simulink model "adrc"  (R2017a)
settings: Solver=FixedStepAuto  StartTime=0.0  StopTime=4  FixedStep=1/30e3  RelTol=1e-3
undefined symbols (not defined in the file): adrc_lib, DiscIntNeverNeededParam, DistObs, h, J, K, Kf, L, R
libraries: simulink_extras x5
settings Model: Creator=uids8840  LastModifiedBy=root

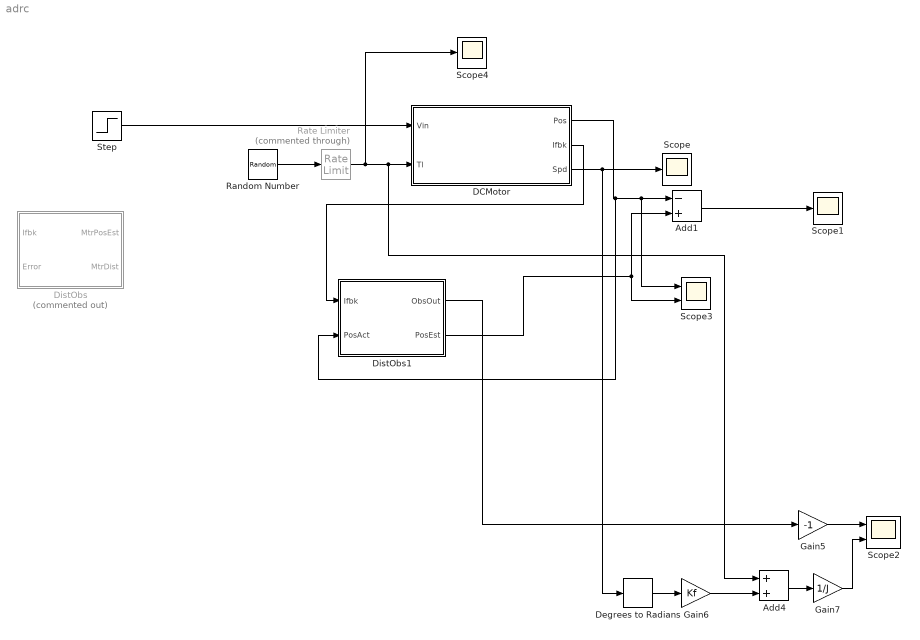
== system adrc ==
  Add1 : Sum  Inputs=-+
  Add4 : Sum
  DCMotor : Subsystem
  Degrees to Radians : simulink_extras/Transformations/Degrees to Radians
  DistObs : Subsystem  Commented=on  SystemSampleTime=1e-3
  DistObs1 : Subsystem  AncestorBlock=adrc_lib/DistObs  TreatAsAtomicUnit=on  SystemSampleTime=1/30e3  mask{k0=-800, k1=-25, k2=-1/4, Jest=J, Kest=K, ts=1/30e3}
      mask prompts: Jest "Motor Inertia [J]"; Kest "Motor Constant [K]"; ts "Execution rate [s]"
  Gain5 : Gain  Gain=-1
  Gain6 : Gain  Gain=Kf
  Gain7 : Gain  Gain=1/J
  Random Number : RandomNumber  Mean=0.03  SampleTime=0.1
  Rate Limiter : RateLimiter  Commented=through  RisingSlewLimit=1e-4  FallingSlewLimit=-1e-4  SampleTimeMode=inherited
  Scope : Scope
  Scope1 : Scope
  Scope2 : Scope  NumInputPorts=2
  Scope3 : Scope  NumInputPorts=2
  Scope4 : Scope
  Step : Step  Time=0.1  After=24  SampleTime=0
  wires:
  Add1/1 -> Scope1/1
  Step/1 -> DCMotor/1(Vin)
  DCMotor/1(Pos) -> DistObs1/2(PosAct), Scope3/1, Add1/1
  Random Number/1 -> Rate Limiter/1
  Add4/1 -> Gain7/1
  Gain7/1 -> Scope2/2
  Gain6/1 -> Add4/2
  Gain5/1 -> Scope2/1
  DistObs1/2(PosEst) -> Scope3/2, Add1/2
  Rate Limiter/1 -> Scope4/1, Add4/1, DCMotor/2(Tl)
  DCMotor/3(Spd) -> Scope/1, Degrees to Radians/1
  DistObs1/1(ObsOut) -> Gain5/1
  DCMotor/2(Ifbk) -> DistObs1/1(Ifbk)
  Degrees to Radians/1 -> Gain6/1

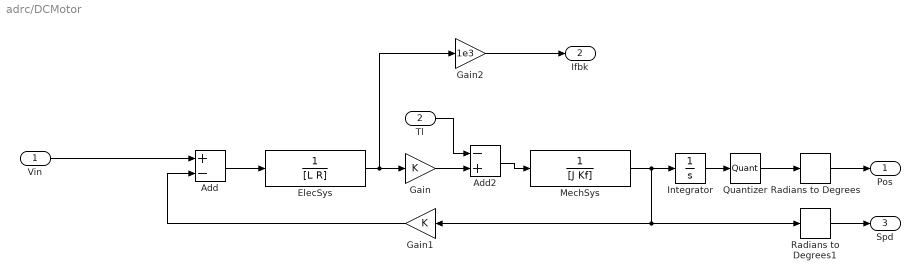
== system adrc/DCMotor ==
  Vin : Inport
  Tl : Inport  Port=2
  Add : Sum  Inputs=+-
  Add2 : Sum  Inputs=-+
  ElecSys : TransferFcn  Denominator=[L R]
  Gain : Gain  Gain=K
  Gain1 : Gain  Gain=K
  Gain2 : Gain  Gain=1e3
  Integrator : Integrator
  MechSys : TransferFcn  Denominator=[J Kf]
  Quantizer : Quantizer  QuantizationInterval=2*pi/400
  Radians to Degrees : simulink_extras/Transformations/Radians to Degrees
  Radians to Degrees1 : simulink_extras/Transformations/Radians to Degrees
  Pos : Outport
  Ifbk : Outport  Port=2
  Spd : Outport  Port=3
  wires:
  Vin/1 -> Add/1
  Gain1/1 -> Add/2
  ElecSys/1 -> Gain2/1, Gain/1
  Integrator/1 -> Quantizer/1
  Gain/1 -> Add2/2
  Add/1 -> ElecSys/1
  Add2/1 -> MechSys/1
  Tl/1 -> Add2/1
  Quantizer/1 -> Radians to Degrees/1
  MechSys/1 -> Radians to Degrees1/1, Gain1/1, Integrator/1
  Radians to Degrees/1 -> Pos/1
  Radians to Degrees1/1 -> Spd/1
  Gain2/1 -> Ifbk/1

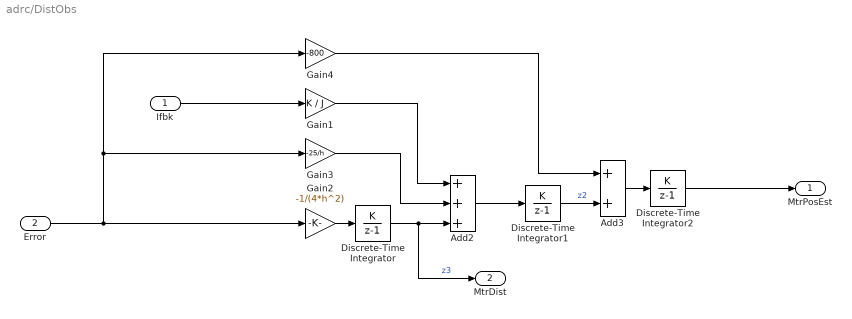
== system adrc/DistObs ==
  Ifbk : Inport
  Error : Inport  Port=2
  Add2 : Sum  Inputs=+++
  Add3 : Sum
  Discrete-Time Integrator : DiscreteIntegrator  IntegratorMethod=Accumulation: Forward Euler  gainval=ts  SampleTime=-1  ICPrevOutput=DiscIntNeverNeededParam  ICPrevScaledInput=DiscIntNeverNeededParam
  Discrete-Time Integrator1 : DiscreteIntegrator  IntegratorMethod=Accumulation: Forward Euler  gainval=ts  SampleTime=-1  ICPrevOutput=DiscIntNeverNeededParam  ICPrevScaledInput=DiscIntNeverNeededParam
  Discrete-Time Integrator2 : DiscreteIntegrator  IntegratorMethod=Accumulation: Forward Euler  gainval=ts  SampleTime=-1  ICPrevOutput=DiscIntNeverNeededParam  ICPrevScaledInput=DiscIntNeverNeededParam
  Gain1 : Gain  Gain=K / J
  Gain2 : Gain  Gain=-1/(4*h^2)
  Gain3 : Gain  Gain=-25/h
  Gain4 : Gain  Gain=-800
  MtrPosEst : Outport
  MtrDist : Outport  Port=2
  wires:
  Discrete-Time Integrator1/1 -> Add3/2  "z2"
  Gain3/1 -> Add2/2
  Add3/1 -> Discrete-Time Integrator2/1
  Discrete-Time Integrator/1 -> MtrDist/1, Add2/3  "z3"
  Gain4/1 -> Add3/1
  Add2/1 -> Discrete-Time Integrator1/1
  Gain1/1 -> Add2/1
  Gain2/1 -> Discrete-Time Integrator/1
  Error/1 -> Gain3/1, Gain4/1, Gain2/1
  Ifbk/1 -> Gain1/1
  Discrete-Time Integrator2/1 -> MtrPosEst/1

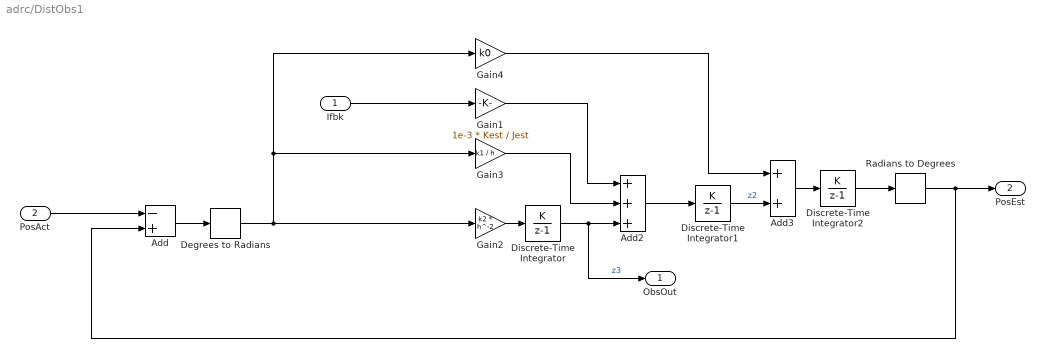
== system adrc/DistObs1 ==
  Ifbk : Inport
  PosAct : Inport  Port=2
  Add : Sum  Inputs=-+
  Add2 : Sum  Inputs=+++
  Add3 : Sum
  Degrees to Radians : simulink_extras/Transformations/Degrees to Radians
  Discrete-Time Integrator : DiscreteIntegrator  IntegratorMethod=Accumulation: Forward Euler  gainval=ts  SampleTime=-1  ICPrevOutput=DiscIntNeverNeededParam  ICPrevScaledInput=DiscIntNeverNeededParam
  Discrete-Time Integrator1 : DiscreteIntegrator  IntegratorMethod=Accumulation: Forward Euler  gainval=ts  SampleTime=-1  ICPrevOutput=DiscIntNeverNeededParam  ICPrevScaledInput=DiscIntNeverNeededParam
  Discrete-Time Integrator2 : DiscreteIntegrator  IntegratorMethod=Accumulation: Forward Euler  gainval=ts  SampleTime=-1  ICPrevOutput=DiscIntNeverNeededParam  ICPrevScaledInput=DiscIntNeverNeededParam
  Gain1 : Gain  Gain=1e-3 * Kest / Jest
  Gain2 : Gain  Gain=k2 * h^-2
  Gain3 : Gain  Gain=k1 / h
  Gain4 : Gain  Gain=k0
  Radians to Degrees : simulink_extras/Transformations/Radians to Degrees
  ObsOut : Outport
  PosEst : Outport  Port=2
  wires:
  Ifbk/1 -> Gain1/1
  Gain2/1 -> Discrete-Time Integrator/1
  Gain1/1 -> Add2/1
  Add2/1 -> Discrete-Time Integrator1/1
  Gain4/1 -> Add3/1
  Discrete-Time Integrator/1 -> Add2/3, ObsOut/1  "z3"
  Add3/1 -> Discrete-Time Integrator2/1
  Gain3/1 -> Add2/2
  Discrete-Time Integrator1/1 -> Add3/2  "z2"
  Add/1 -> Degrees to Radians/1
  PosAct/1 -> Add/1
  Discrete-Time Integrator2/1 -> Radians to Degrees/1
  Radians to Degrees/1 -> Add/2, PosEst/1
  Degrees to Radians/1 -> Gain2/1, Gain4/1, Gain3/1
